simulink model "lab3"  (R2018a)
settings: Solver=VariableStepAuto  StartTime=0.0  StopTime=0.04  RelTol=1e-3
libraries: powerlib x11, powerlib_meascontrol x4
settings Model: Creator=Aniket Raj  LastModifiedBy=Aniket Raj

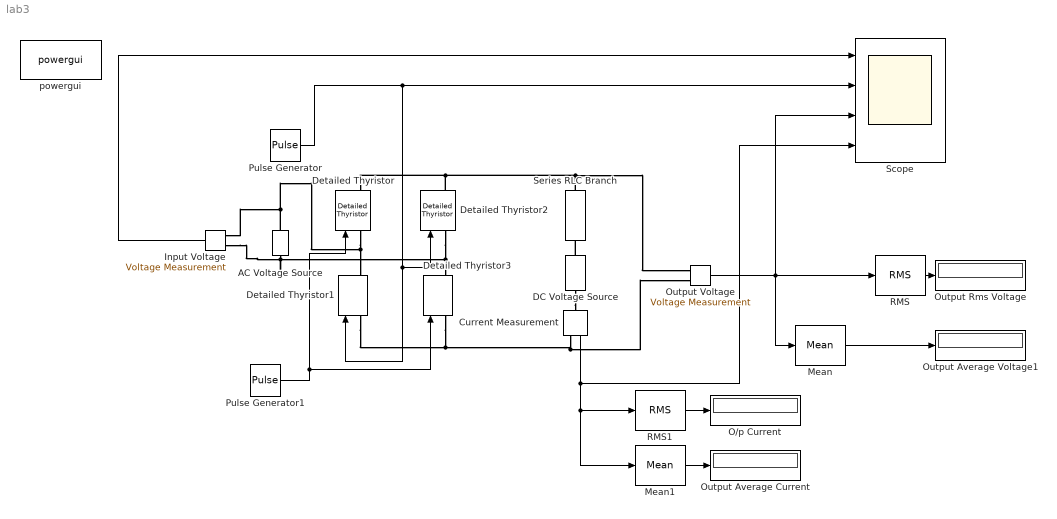
== system lab3 ==
  AC Voltage Source : powerlib/Electrical Sources/AC Voltage Source  Amplitude=230  Phase=0  Frequency=50  SampleTime=0  Measurements=None  BusType=swing  Pref=10e3  Qref=0  Qmin=-inf  Qmax=+inf
  Current Measurement : powerlib/Measurements/Current Measurement  PhasorSimulation=off  OutputType=Complex  PSBequivalent=0
  DC Voltage Source : powerlib/Electrical Sources/DC Voltage Source  Amplitude=48  Measurements=None
  Detailed Thyristor{,1..3} (4 alike) : powerlib/Power Electronics/Detailed Thyristor  Ron=0.001  Lon=1e-3  Vf=0.8  IL=0.1  Tq=100e-6  IC=0  Rs=500  Cs=250e-9  Measurements=on
      settings: SourceProductName=Simscape Power Systems  SourceProductBaseCode=PS
  "Input Voltage " : powerlib/Measurements/Voltage Measurement  PhasorSimulation=off  OutputType=Complex  PSBequivalent=0
  Mean : powerlib_meascontrol/Measurements/Mean  Freq=50  Vinit=0  Ts=0
  Mean1 : powerlib_meascontrol/Measurements/Mean  Freq=50  Vinit=0  Ts=0
  "O/p Current " : Display
  Output Average Current : Display
  Output Average Voltage1 : Display
  Output Rms Voltage : Display
  "Output Voltage " : powerlib/Measurements/Voltage Measurement  PhasorSimulation=off  OutputType=Complex  PSBequivalent=0
  Pulse Generator : DiscretePulseGenerator  PulseType=Time based  Period=0.02  PulseWidth=0.1  PhaseDelay=0.01+(0.02/360)*60
  Pulse Generator1 : DiscretePulseGenerator  PulseType=Time based  Period=0.02  PulseWidth=0.1  PhaseDelay=(0.02/360)*60
  RMS : powerlib_meascontrol/Measurements/RMS  TrueRMS=on  Freq=50  RMSInit=120  Ts=0
  RMS1 : powerlib_meascontrol/Measurements/RMS  TrueRMS=on  Freq=50  RMSInit=120  Ts=0
  Scope : Scope  NumInputPorts=4
  Series RLC Branch : powerlib/Elements/Series RLC Branch  LConnTagsString=__new0  RConnTagsString=__new0  BranchType=RL  Resistance=1  Inductance=0.002  SetiL0=off  InitialCurrent=0  Capacitance=1e-6  Setx0=off  InitialVoltage=0  Measurements=None
  powergui : powerlib/powergui  Priority=1  SimulationMode=Continuous  SampleTime=50e-6  frequency=60  Iterations=50  frequencyindice=50  Pbase=100e6  ErrMax=1e-4  UnitsV=kV  UnitsW=MW  buscounter=0  FunctionMessages=off  echomessages=off  EnableUseOfTLC=off  CurrentSourceSwitches=off  DisableSnubberDevices=off  DisableRonSwitches=off  DisableVfSwitches=off  DisplayEquations=off  SolverType=Tustin/Backward Euler (TBE)  Interpol=off  ExternalGateDelay=off  methode=off  Ts=100  x0status=blocks  SPID=on  SwTol=0  HookPort=off  RestoreLinks=warning  ResistiveCurrentMeasurement=off  Frange=[0:2:500]  Ylog=off  Xlog=on  ShowGrid=off  save=off  variable=ZData  structure=0  ZoomFFT=off  StartTime=0.0  cycles=1  DisplayStyle=1  fundamental=60  FreqAxis=off  MaxFrequency=1000  frequencyindicesteady=1  RmsSteady=1  display=off
  wires:
  "Input Voltage "/1 -> Scope/1
  "Output Voltage "/1 -> Mean/1, RMS/1, Scope/3
  RMS/1 -> Output Rms Voltage/1
  Mean/1 -> Output Average Voltage1/1
  Current Measurement/1 -> Scope/4, Mean1/1, RMS1/1
  RMS1/1 -> "O/p Current "/1
  Mean1/1 -> Output Average Current/1
  Pulse Generator/1 -> Detailed Thyristor1/1, Detailed Thyristor2/1, Scope/2
  Pulse Generator1/1 -> Detailed Thyristor3/1, Detailed Thyristor/1
  connections:
  Current Measurement/RConn1 -- Detailed Thyristor3/LConn1 -- Detailed Thyristor1/LConn1 -- "Output Voltage "/LConn2
  Series RLC Branch/LConn1 -- Detailed Thyristor2/RConn1 -- Detailed Thyristor/RConn1 -- "Output Voltage "/LConn1
  DC Voltage Source/LConn1 -- Current Measurement/LConn1
  DC Voltage Source/RConn1 -- Series RLC Branch/RConn1
  Detailed Thyristor/LConn1 -- "Input Voltage "/LConn1 -- AC Voltage Source/RConn1 -- Detailed Thyristor1/RConn1
  Detailed Thyristor2/LConn1 -- "Input Voltage "/LConn2 -- AC Voltage Source/LConn1 -- Detailed Thyristor3/RConn1
